simulink model "part1_h"  (R2023b)
settings: Solver=VariableStepAuto  StartTime=0.0  StopTime=50  RelTol=1e-3
settings Model: Creator=setarehdehghanfard
settings DebuggingCC: UnconnectedInputMsg=warning  UnconnectedOutputMsg=warning  UnconnectedLineMsg=warning
settings ModelReferenceCC: EnableRefExpFcnMdlSchedulingChecks=on
settings RTWCC: DLArmComputeVersion=19.05

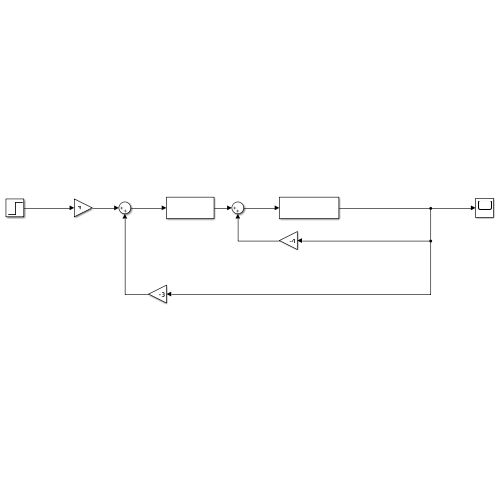
[thumbnail: Simulink's stored preview of the top-level diagram]
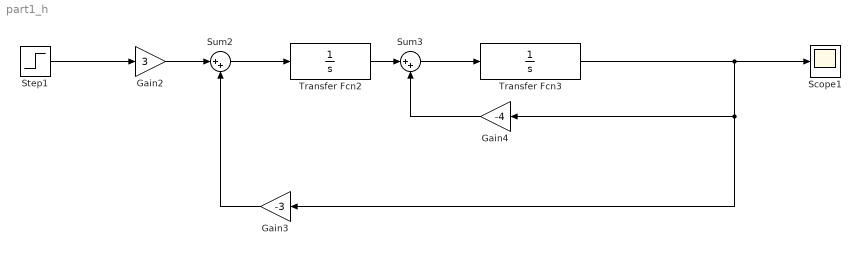
== system part1_h ==
  Gain2 : Gain  Gain=3
  Gain3 : Gain  Gain=-3
  Gain4 : Gain  Gain=-4
  Scope1 : Scope
  Step1 : Step  SampleTime=0
  Sum2 : Sum  Inputs=|++
  Sum3 : Sum  Inputs=|++
  Transfer Fcn2 : TransferFcn  Denominator=[1 0]
  Transfer Fcn3 : TransferFcn  Denominator=[1 0]
  wires:
  Sum2/1 -> Transfer Fcn2/1
  Sum3/1 -> Transfer Fcn3/1
  Transfer Fcn2/1 -> Sum3/1
  Gain2/1 -> Sum2/1
  Gain3/1 -> Sum2/2
  Gain4/1 -> Sum3/2
  Transfer Fcn3/1 -> Scope1/1, Gain3/1, Gain4/1
  Step1/1 -> Gain2/1
